simulink model "torque_controller"  (R2015a)
settings: Solver=FixedStepDiscrete  StartTime=0.0  StopTime=inf  FixedStep=sample_time  RelTol=1e-3
StartFcn:
  | tg.sampletime = correctedSampleTime;
settings Model: SimulationMode=external  CovSFcnEnable=off  Creator=wmartin  LastModifiedBy=robots
settings SolverCC: EnableConcurrentExecution=on
settings DataIOCC: LimitDataPoints=off  MaxDataPoints=1e7  SaveFormat=StructureWithTime  SignalLogging=off  DSMLogging=off
settings OptimizationCC: BlockReduction=off  OptimizeBlockIOStorage=off  BufferReuse=off  GlobalBufferReuse=off  ExpressionFolding=off  ExpressionDepthLimit=2147483647  LocalBlockOutputs=off  SimCompilerOptimization=on
settings DebuggingCC: UnderspecifiedInitializationDetection=Classic  MergeDetectMultiDrivingBlocksExec=none  SolverPrmCheckMsg=warning  StateNameClashWarn=warning
settings HardwareCC: ProdIntDivRoundTo=Zero  ProdEndianess=LittleEndian  ProdLongLongMode=on  ProdHWDeviceType=Generic->32-bit x86 compatible
settings ModelReferenceCC: UpdateModelReferenceTargets=IfOutOfDate  ModelReferenceNumInstancesAllowed=Single  ModelReferenceMinAlgLoopOccurrences=on
settings RTWCC: SystemTargetFile=slrt.tlc  TemplateMakefile=slrt_default_tmf  Description=Simulink Real-Time  RTWVerbose=off  RTWCompilerOptimization=on
settings CodeAppCC: MaxIdLength=256
settings SimulinkRealTimeCC: GeneratePreprocessorConditionals=Disable all  RL32LogBufSizeModifier=1e8

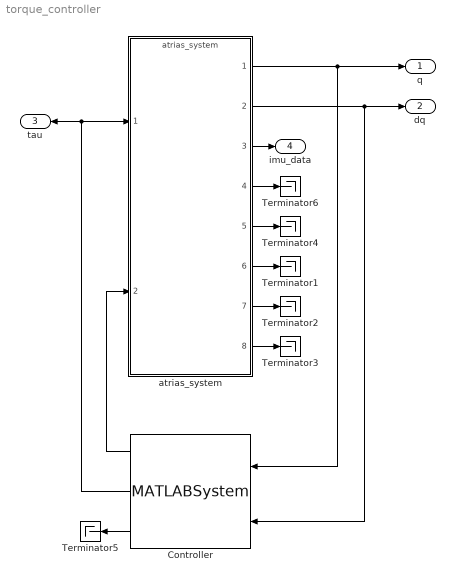
== system torque_controller ==
  Controller : MATLABSystem  System=TorqueController  isSim=off  ps3Axes=[0 0 0 0]  ps3Buttons=[0 0 0 0 0 0 0 0 0 0 0 0 0 0 0 0 0]  u_lim=50  SimulateUsing=Code generation
      mask Type: TorqueController
      mask Display:
      | disp('TorqueController');
      | port_label('input',1,'q');
      | port_label('input',2,'dq');
      | port_label('output',1,'eStop');
      | port_label('output',2,'u');
      | port_label('output',3,'userOut');
  Terminator{1..6} (6 alike) : Terminator
  atrias_system : ModelReference  ModelNameDialog=atrias_system  SimulationMode=Normal  ModelReferenceVersion=1.2753  CopyOfModelName=atrias_system  DefaultDataLogging=on
  q : Outport
  dq : Outport  Port=2
  tau : Outport  Port=3
  imu_data : Outport  Port=4
  wires:
  atrias_system/2 -> dq/1, Controller/2
  atrias_system/1 -> Controller/1, q/1
  atrias_system/6 -> Terminator1/1
  atrias_system/7 -> Terminator2/1
  atrias_system/8 -> Terminator3/1
  atrias_system/3 -> imu_data/1
  Controller/2 -> atrias_system/1, tau/1
  Controller/1 -> atrias_system/2
  Controller/3 -> Terminator5/1
  atrias_system/5 -> Terminator4/1
  atrias_system/4 -> Terminator6/1
